simulink model "Controllo_Adattativo"  (R2023a)
settings: Solver=VariableStepAuto  StartTime=0.0  StopTime=113  RelTol=1e-3
values from neighbouring files (symbols this model uses):
  a1 = 0.5    [Progetto_FoR.m]
  d0 = 1    [Progetto_FoR.m]
  KD = diag(kd)    [Progetto_FoR.m]
  KD3 = diag(kd3)    [Progetto_FoR.m]
  KP = diag(kp)    [Progetto_FoR.m]
  Lambda = diag(lambda)    [Progetto_FoR.m]
  pi0 = [ml1 Il1 Im1 Fm1 ml2 Il2 Im2 Fm2 ml3 Im3 Fm3 Il4 Im4 Fm4]    [Progetto_FoR.m]
  q0 = [0 pi/2 0 pi/2]    [Progetto_FoR.m]
  Tc = 0.001    [Progetto_FoR.m]
undefined symbols (not defined in the file or in its folder): DiscIntNeverNeededParam
settings Model: Creator=panto  LastModifiedBy=panto

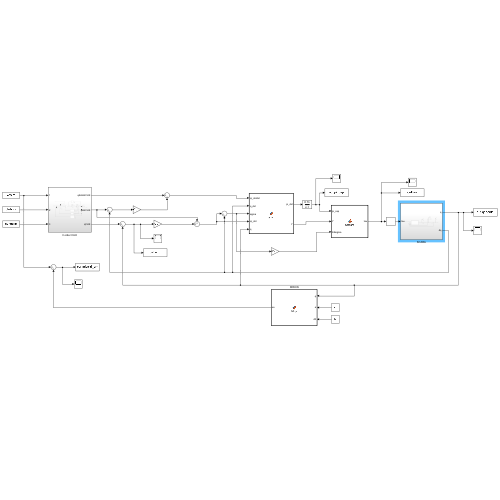
[thumbnail: Simulink's stored preview of the top-level diagram]
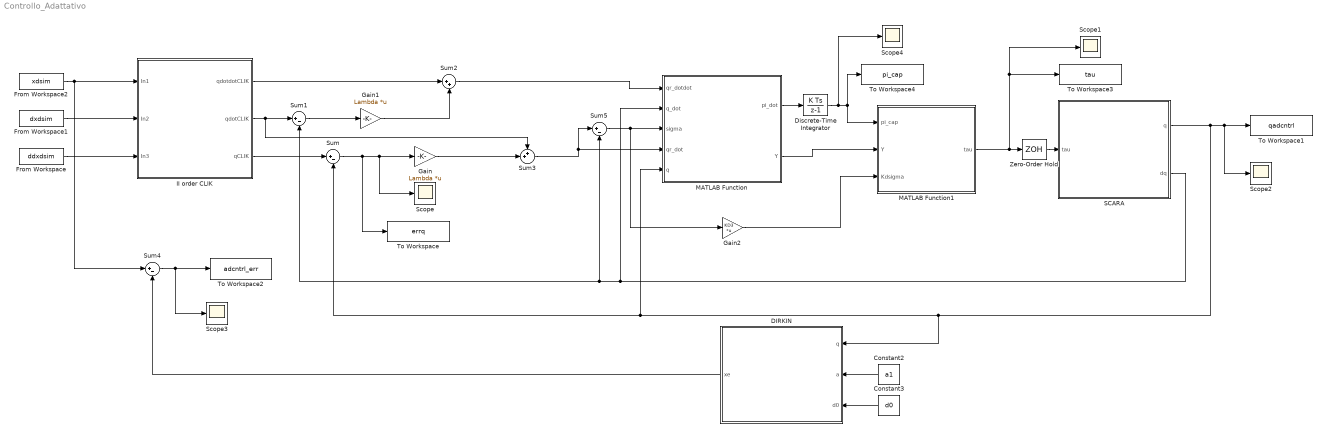
== system Controllo_Adattativo ==
  Constant2 : Constant  Value=a1
  Constant3 : Constant  Value=d0
  DIRKIN : MATLAB Function  TreatAsAtomicUnit=on
  Discrete-Time Integrator : DiscreteIntegrator  InitialCondition=pi0'  SampleTime=-1  ICPrevOutput=DiscIntNeverNeededParam  ICPrevScaledInput=DiscIntNeverNeededParam
  From Workspace : FromWorkspace  VariableName=ddxdsim  SampleTime=Tc
  From Workspace1 : FromWorkspace  VariableName=dxdsim  SampleTime=Tc
  From Workspace2 : FromWorkspace  VariableName=xdsim  SampleTime=Tc
  Gain : Gain  Gain=Lambda  Multiplication=Matrix(K*u)
  Gain1 : Gain  Gain=Lambda  Multiplication=Matrix(K*u)
  Gain2 : Gain  Gain=KD3  Multiplication=Matrix(K*u)
  II order CLIK : Subsystem
  MATLAB Function : MATLAB Function  TreatAsAtomicUnit=on
  MATLAB Function1 : MATLAB Function  TreatAsAtomicUnit=on
  SCARA : Subsystem
  Scope{,1..4} (5 alike) : Scope
  Sum{,1,4..5} (4 alike) : Sum  Inputs=|+-
  Sum2 : Sum  Inputs=|++
  Sum3 : Sum  Inputs=++|
  To Workspace : ToWorkspace  VariableName=errq  SampleTime=Tc
      settings: Save2DSignal=2-D array (concatenate along first dimension)
  To Workspace1 : ToWorkspace  VariableName=qadcntrl  SampleTime=-1
      settings: Save2DSignal=2-D array (concatenate along first dimension)
  To Workspace2 : ToWorkspace  VariableName=adcntrl_err  SampleTime=Tc
      settings: Save2DSignal=2-D array (concatenate along first dimension)
  To Workspace3 : ToWorkspace  VariableName=tau  SampleTime=-1
      settings: Save2DSignal=2-D array (concatenate along first dimension)
  To Workspace4 : ToWorkspace  VariableName=pi_cap  SampleTime=-1
      settings: Save2DSignal=2-D array (concatenate along first dimension)
  Zero-Order Hold : ZeroOrderHold  SampleTime=-1
  wires:
  From Workspace1/1 -> II order CLIK/2(In2)
  From Workspace2/1 -> Sum4/1, II order CLIK/1(In1)
  From Workspace/1 -> II order CLIK/3(In3)
  DIRKIN/1(xe) -> Sum4/2
  Constant2/1 -> DIRKIN/2(a)
  Constant3/1 -> DIRKIN/3(d0)
  MATLAB Function1/1(tau) -> Zero-Order Hold/1, Scope1/1, To Workspace3/1
  II order CLIK/3(qCLIK) -> Sum/1
  II order CLIK/1(qdotdotCLIK) -> Sum2/1
  II order CLIK/2(qdotCLIK) -> Sum3/1, Sum1/1
  Sum/1 -> To Workspace/1, Scope/1, Gain/1
  Sum1/1 -> Gain1/1
  Gain1/1 -> Sum2/2
  Gain/1 -> Sum3/2
  SCARA/1(q) -> To Workspace1/1, Scope2/1, DIRKIN/1(q), MATLAB Function/5(q), Sum/2
  SCARA/2(dq) -> Sum5/2, Sum1/2, MATLAB Function/2(q_dot)
  Sum4/1 -> Scope3/1, To Workspace2/1
  Sum2/1 -> MATLAB Function/1(qr_dotdot)
  Sum3/1 -> Sum5/1, MATLAB Function/4(qr_dot)
  Sum5/1 -> Gain2/1, MATLAB Function/3(sigma)
  MATLAB Function/2(Y) -> MATLAB Function1/2(Y)
  Gain2/1 -> MATLAB Function1/3(Kdsigma)
  MATLAB Function/1(pi_dot) -> Discrete-Time Integrator/1
  Discrete-Time Integrator/1 -> Scope4/1, To Workspace4/1, MATLAB Function1/1(pi_cap)
  Zero-Order Hold/1 -> SCARA/1(tau)

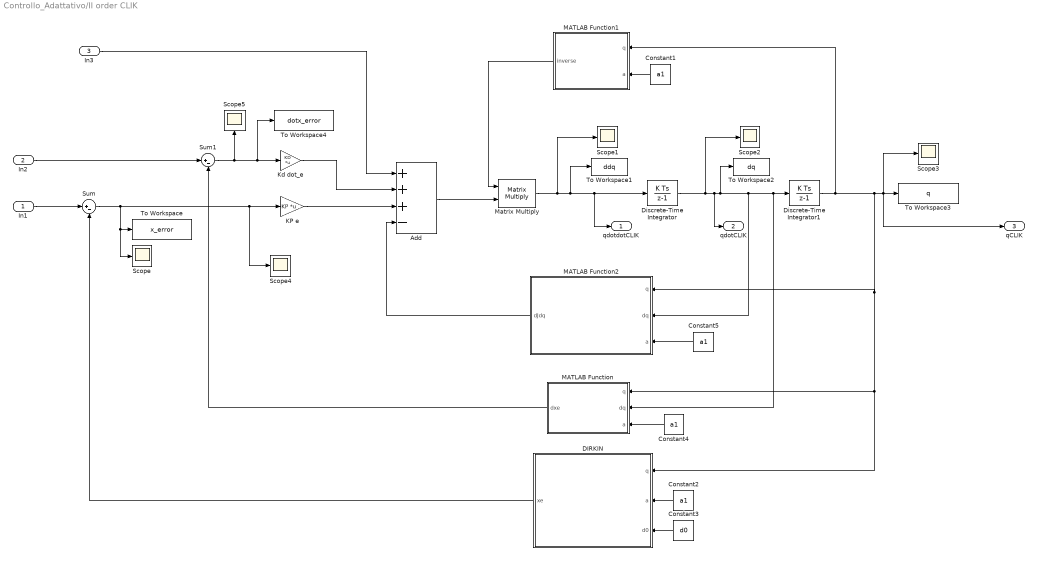
== system Controllo_Adattativo/II order CLIK ==
  In1 : Inport
  In2 : Inport  Port=2
  In3 : Inport  Port=3
  Add : Sum  Inputs=+++-
  Constant{1..2,4..5} (4 alike) : Constant  Value=a1
  Constant3 : Constant  Value=d0
  DIRKIN : MATLAB Function  TreatAsAtomicUnit=on
  Discrete-Time Integrator : DiscreteIntegrator  InitialCondition=[0;0;0;0]  SampleTime=Tc  ICPrevOutput=DiscIntNeverNeededParam  ICPrevScaledInput=DiscIntNeverNeededParam
  Discrete-Time Integrator1 : DiscreteIntegrator  InitialCondition=q0'  SampleTime=Tc  ICPrevOutput=DiscIntNeverNeededParam  ICPrevScaledInput=DiscIntNeverNeededParam
  KP e : Gain  Gain=KP  Multiplication=Matrix(K*u)
  Kd dot_e : Gain  Gain=KD  Multiplication=Matrix(K*u)
  MATLAB Function : MATLAB Function  TreatAsAtomicUnit=on
  MATLAB Function1 : MATLAB Function  TreatAsAtomicUnit=on
  MATLAB Function2 : MATLAB Function  TreatAsAtomicUnit=on
  Matrix Multiply : Product  Multiplication=Matrix(*)
  Scope{,1..5} (6 alike) : Scope
  Sum : Sum  Inputs=|+-
  Sum1 : Sum  Inputs=|+-
  To Workspace : ToWorkspace  VariableName=x_error  SampleTime=Tc
      settings: Save2DSignal=2-D array (concatenate along first dimension)
  To Workspace1 : ToWorkspace  VariableName=ddq  SampleTime=-1
      settings: Save2DSignal=2-D array (concatenate along first dimension)
  To Workspace2 : ToWorkspace  VariableName=dq  SampleTime=-1
      settings: Save2DSignal=2-D array (concatenate along first dimension)
  To Workspace3 : ToWorkspace  VariableName=q  SampleTime=Tc
      settings: Save2DSignal=2-D array (concatenate along first dimension)
  To Workspace4 : ToWorkspace  VariableName=dotx_error  SampleTime=-1
      settings: Save2DSignal=2-D array (concatenate along first dimension)
  qdotdotCLIK : Outport
  qdotCLIK : Outport  Port=2
  qCLIK : Outport  Port=3
  wires:
  Discrete-Time Integrator/1 -> Scope2/1, qdotCLIK/1, To Workspace2/1, MATLAB Function2/2(dq), MATLAB Function/2(dq), Discrete-Time Integrator1/1
  Sum/1 -> Scope/1, To Workspace/1, Scope4/1, KP e/1
  Kd dot_e/1 -> Add/2
  In2/1 -> Sum1/1
  Constant5/1 -> MATLAB Function2/3(a)
  Constant1/1 -> MATLAB Function1/2(a)
  Constant3/1 -> DIRKIN/3(d0)
  KP e/1 -> Add/3
  Matrix Multiply/1 -> Scope1/1, To Workspace1/1, qdotdotCLIK/1, Discrete-Time Integrator/1
  MATLAB Function/1(dxe) -> Sum1/2
  Constant4/1 -> MATLAB Function/3(a)
  Add/1 -> Matrix Multiply/2
  In3/1 -> Add/1
  Discrete-Time Integrator1/1 -> MATLAB Function2/1(q), MATLAB Function/1(q), DIRKIN/1(q), qCLIK/1, Scope3/1, To Workspace3/1, MATLAB Function1/1(q)
  In1/1 -> Sum/1
  MATLAB Function2/1(dJdq) -> Add/4
  DIRKIN/1(xe) -> Sum/2
  Constant2/1 -> DIRKIN/2(a)
  MATLAB Function1/1(inverse) -> Matrix Multiply/1
  Sum1/1 -> Scope5/1, To Workspace4/1, Kd dot_e/1

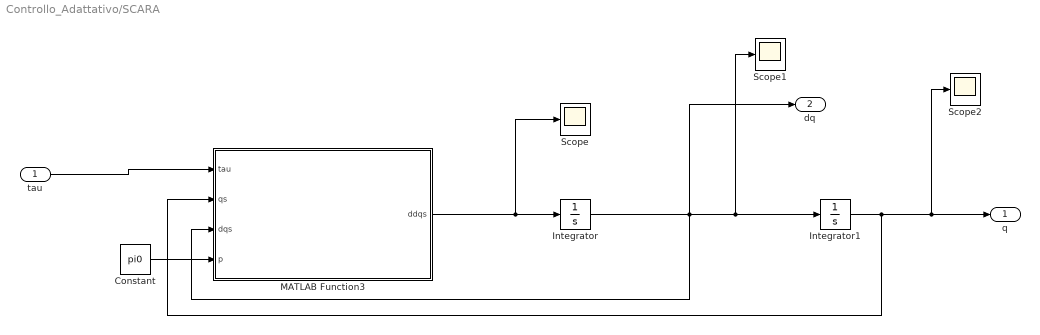
== system Controllo_Adattativo/SCARA ==
  tau : Inport
  Constant : Constant  Value=pi0
  Integrator : Integrator  InitialCondition=[0;0;0;0]
  Integrator1 : Integrator  InitialCondition=q0'
  MATLAB Function3 : MATLAB Function  TreatAsAtomicUnit=on
  Scope : Scope
  Scope1 : Scope
  Scope2 : Scope
  q : Outport  SampleTime=Tc
  dq : Outport  Port=2  SampleTime=Tc
  wires:
  Integrator/1 -> dq/1, MATLAB Function3/3(dqs), Integrator1/1, Scope1/1
  tau/1 -> MATLAB Function3/1(tau)
  Integrator1/1 -> MATLAB Function3/2(qs), Scope2/1, q/1
  MATLAB Function3/1(ddqs) -> Integrator/1, Scope/1
  Constant/1 -> MATLAB Function3/4(p)

== matlab function Controllo_Adattativo/II order CLIK/MATLAB Function1 ==
  data: q input; inverse output; a input
function inverse = invJ(q,a)
%devo prima calcolare lo Jacobiano analitico e poi invertirlo
%Nel caso dello SCARA, lo Jacobiano analitico coincide con quello
%geometrico: questo perchè nello SCARA l'orientamento può essere
%rappresentato direttamente dall'angolo attorno a z, e quindi la velocità
%angolare z si traduce direttamente nella velocità di cambiamento
%dell'angolo di orientamento attorno z
%dal libro when the DOFs cause rotations of the end-effector all about the 
% same fixed axis in space, the two Jacobians are essentially the same
   
    Ja = zeros(4,4);
    Ja = [-a*sin(q(1)+q(2))-a*sin(q(1)) -a*sin(q(1)+q(2)) 0 0;
        a*cos(q(1)+q(2))+a*cos(q(1)) a*cos(q(1)+q(2)) 0 0;
        0 0 -1 0;
        1 1 0 -1];

    inverse = inv(Ja);

end

== matlab function Controllo_Adattativo/II order CLIK/DIRKIN ==
  data: q input; xe output; a input; d0 input
function xe = dirkyn(q, a, d0)
  xe = zeros(4,1);
    xe = [a*cos(q(1)+q(2))+a*cos(q(1));
        a*sin(q(1)+q(2))+a*sin(q(1));
        d0-q(3);
        q(1)+q(2)-q(4)];
end

== matlab function Controllo_Adattativo/II order CLIK/MATLAB Function ==
  data: q input; dq input; dxe output; a input
function dxe = Ja(q,dq,a)

Ja = zeros(4,4);
Ja = [-a*sin(q(1)+q(2))-a*sin(q(1)) -a*sin(q(1)+q(2)) 0 0;
        a*cos(q(1)+q(2))+a*cos(q(1)) a*cos(q(1)+q(2)) 0 0;
        0 0 -1 0;
        1 1 0 -1];

    dxe = Ja*dq;

end

== matlab function Controllo_Adattativo/II order CLIK/MATLAB Function2 ==
  data: q input; dq input; dJdq output; a input
function dJdq =  dotJadotq(q,dq,a)
    
    dotJa = zeros(4,4);
    dotJa = [-a*cos(q(1))*dq(1)-a*cos(q(1)+q(2))*(dq(1)+dq(2)) -a*cos(q(1)+q(2))*(dq(1)+dq(2)) 0 0;
        -a*sin(q(1))*dq(1)-a*sin(q(1)+q(2))*(dq(1)+dq(2)) -a*sin(q(1)+q(2))*(dq(1)+dq(2)) 0 0;
        0 0 0 0;
        0 0 0 0];

    dJdq = dotJa*dq;

end

== matlab function Controllo_Adattativo/DIRKIN ==
  data: q input; xe output; a input; d0 input
function xe = dirkyn(q, a, d0)
  xe = zeros(4,1);
    xe = [a*cos(q(1)+q(2))+a*cos(q(1));
        a*sin(q(1)+q(2))+a*sin(q(1));
        d0-q(3);
        q(1)+q(2)-q(4)];
end

== matlab function Controllo_Adattativo/MATLAB Function ==
  data: pi_dot output; qr_dotdot input; q_dot input; sigma input; qr_dot input; q input; Y output
function [pi_dot, Y] = param(qr_dotdot, q_dot, sigma, qr_dot, q)

%Y è data dalla derivata rispetto ai parametri di B*qr_dotdot + C*qr_dot +
%F_v*qr_dot + g, quindi, su carta e penna, calcolo prima i prodotti, poi le
%derivate e poi sommo le matrici derivate, e ottengo cosi la matrice dei
%regressori; definisco quindi le matrici derivate
Fv_der = zeros(4,14);
Fv_der(1,4) = qr_dot(1);
Fv_der(2,8) = qr_dot(2);
Fv_der(3,11) = 2500*qr_dot(3);
Fv_der(4,14) = 400*qr_dot(4);

C_der = zeros(4,14);
C_der(1,5) = -0.125*sin(q(2))*(q_dot(2)*qr_dot(1)+qr_dot(2)*(q_dot(1)+q_dot(2)));
C_der(1,9) = -0.25*sin(q(2))*(q_dot(2)*qr_dot(1)+qr_dot(2)*(q_dot(1)+q_dot(2)));
C_der(2,5) = 0.125*sin(q(2))*(q_dot(1)*qr_dot(1));
C_der(2,9) = 0.25*sin(q(2))*(q_dot(1)*qr_dot(1));

B_der = zeros(4,14);
B_der(1,1) = 0.125*qr_dotdot(1);
B_der(1,2) = qr_dotdot(1);
B_der(1,3) = qr_dotdot(1);
B_der(1,5) = qr_dotdot(1)*(0.25+0.125+0.25*cos(q(2))) + qr_dotdot(2)*(0.125+0.125*cos(q(2)));
B_der(1,6) = qr_dotdot(1) + qr_dotdot(2);
B_der(1,9) = qr_dotdot(1)*(0.5+0.5*cos(q(2))) + qr_dotdot(2)*(0.25+0.25*cos(q(2)));
B_der(1,12) = qr_dotdot(1) + qr_dotdot(2) - qr_dotdot(4);
B_der(2,5) = qr_dotdot(1)*(0.125+0.125*cos(q(2))) + qr_dotdot(2)*0.125;
B_der(2,6) = qr_dotdot(1) + qr_dotdot(2);
B_der(2,7) = qr_dotdot(2);
B_der(2,9) = qr_dotdot(1)*(0.25+0.25*cos(q(2))) + 0.25*qr_dotdot(2);
B_der(2,12) = qr_dotdot(1) + qr_dotdot(2) - qr_dotdot(4);
B_der(3,9) = qr_dotdot(3);
B_der(3,10) = qr_dotdot(3)*2500;
B_der(4,12) = qr_dotdot(4) - qr_dotdot(1) - qr_dotdot(2);
B_der(4,13) = qr_dotdot(4)*400;

g_der = zeros(4,14);
g_der(3,9) = -9.81;

Y = B_der + C_der + Fv_der + g_der;

% Definire la matrice Kpi
kpi = [100 100 100 100 100 100 100 100 0.01 100 100 100 100 100];
Kpi = diag(kpi);

% Calcolare pi_dot
pi_dot = Kpi\ Y' * sigma;

end

== matlab function Controllo_Adattativo/MATLAB Function1 ==
  data: pi_cap input; Y input; tau output; Kdsigma input
function tau = ingresso(pi_cap,Y,Kdsigma)

tau = Y*pi_cap + Kdsigma;

end

== matlab function Controllo_Adattativo/SCARA/MATLAB Function3 ==
  data: tau input; ddqs output; qs input; dqs input; p input
function ddqs = SCARA(tau,qs,dqs,p)
   %devo implementare l'equazione ddq = B^-1 (tau-tau')
    %inizio calcolando B
    b11 = p(2)+p(6)+p(12)+p(1)*0.0625+p(5)*(0.25+0.0625+0.25*cos(qs(2))) + p(9)*(0.5+0.5*cos(qs(2)))+p(3);
    b22 = p(6) + p(12) + p(5)*0.0625 + p(9)*0.25 + p(7);
    b33 = p(9) +2500*p(10);
    b44 = p(12) + 400*p(13);
    b12 = p(2) + p(12) + p(5)*(0.0625+0.125*cos(qs(2))) + p(9)*(0.25+0.25*cos(qs(2)));
    b21 = b12;
    b14 = -p(12);
    b41 = b14;
    b24 = b14;
    b42 = b14;
    
    B = [b11 b12 0 b14;
        b21 b22 0 b24;
        0 0 b33 0;
        b41 b42 0 b44];
    %poi mi servono C, Fv e gravità

    k = -p(5)*0.125*sin(qs(2)) - p(9)*0.25*sin(qs(2)); %costante per la matrice C
    gr = 9.81;
    mp = 3; %Payload
    g = [0; 0; -gr*(p(9)+mp); 0];

    %Matrice degli attriti viscosi
    f_v = [0.00005 0.00005 25 2];
    F_v = diag(f_v);

    C = [k*dqs(2) k*(dqs(1)+dqs(2)) 0 0;
         -k*dqs(1) 0 0 0;
            0 0 0 0;
            0 0 0 0];
    
    tau_primo = C*dqs+F_v*dqs +g;
   
    ddqs = inv(B)*(tau-tau_primo);



end
